simulink model "pi_IL_H2DF_2024a"  (R2024a)
settings: Solver=FixedStepAuto  StartTime=0.0  StopTime=inf  FixedStep=0.001  RelTol=1e-3  EnableMultiTasking=on
values from neighbouring files (symbols this model uses):
  IL = struct()    [init_simulink_IL_H2DF.m]
undefined symbols (not defined in the file or in its folder): C2C_NMPC
libraries: deeplib x1, raspberrypiNetworklib x1
(part 2 of 2)

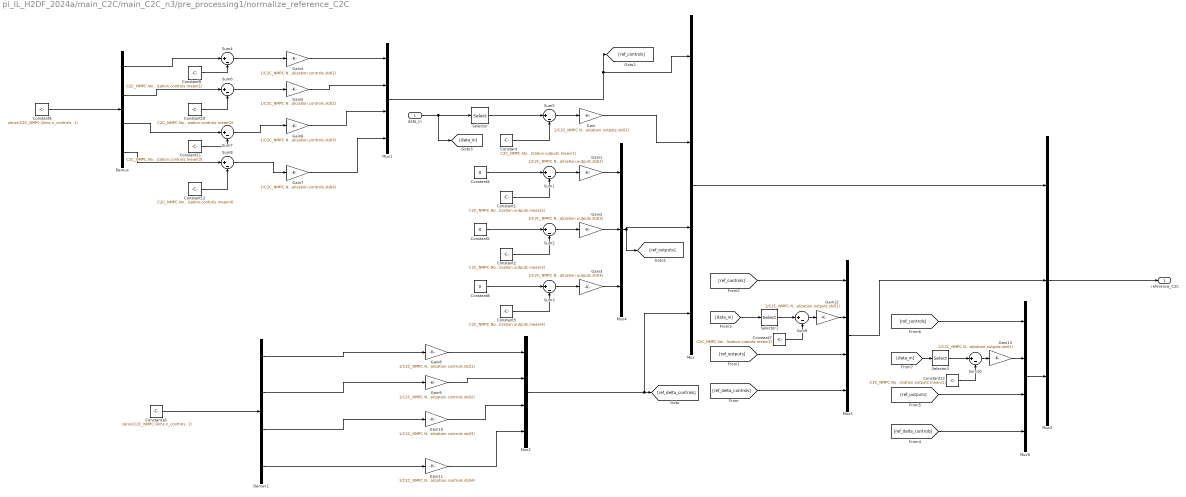
== system pi_IL_H2DF_2024a/main_C2C/main_C2C_n3/pre_processing1/normalize_reference_C2C ==
  data_in : Inport
  Constant : Constant  Value=C2C_NMPC.Normalization.outputs.mean(1)
  Constant1 : Constant  Value=C2C_NMPC.Normalization.outputs.mean(2)
  Constant10 : Constant  Value=C2C_NMPC.Normalization.controls.mean(2)
  Constant11 : Constant  Value=C2C_NMPC.Normalization.controls.mean(3)
  Constant12 : Constant  Value=C2C_NMPC.Normalization.controls.mean(4)
  Constant13 : Constant  Value=C2C_NMPC.Normalization.outputs.mean(1)
  Constant16 : Constant  Value=zeros(C2C_NMPC.Dims.n_controls, 1)
  Constant2 : Constant  Value=C2C_NMPC.Normalization.outputs.mean(3)
  Constant3 : Constant  Value=C2C_NMPC.Normalization.outputs.mean(4)
  Constant4 : Constant  Value=0
  Constant5 : Constant  Value=0
  Constant6 : Constant  Value=zeros(C2C_NMPC.Dims.n_controls, 1)
  Constant7 : Constant  Value=C2C_NMPC.Normalization.outputs.mean(1)
  Constant8 : Constant  Value=0
  Constant9 : Constant  Value=C2C_NMPC.Normalization.controls.mean(1)
  Demux : Demux
  Demux1 : Demux
  Gain : Gain  Gain=1/C2C_NMPC.Normalization.outputs.std(1)
  Gain1 : Gain  Gain=1/C2C_NMPC.Normalization.outputs.std(2)
  Gain10 : Gain  Gain=1/C2C_NMPC.Normalization.controls.std(3)
  Gain11 : Gain  Gain=1/C2C_NMPC.Normalization.controls.std(4)
  Gain12 : Gain  Gain=1/C2C_NMPC.Normalization.outputs.std(1)
  Gain13 : Gain  Gain=1/C2C_NMPC.Normalization.outputs.std(1)
  Gain2 : Gain  Gain=1/C2C_NMPC.Normalization.outputs.std(3)
  Gain3 : Gain  Gain=1/C2C_NMPC.Normalization.outputs.std(4)
  Gain4 : Gain  Gain=1/C2C_NMPC.Normalization.controls.std(1)
  Gain5 : Gain  Gain=1/C2C_NMPC.Normalization.controls.std(2)
  Gain6 : Gain  Gain=1/C2C_NMPC.Normalization.controls.std(3)
  Gain7 : Gain  Gain=1/C2C_NMPC.Normalization.controls.std(4)
  Gain8 : Gain  Gain=1/C2C_NMPC.Normalization.controls.std(1)
  Gain9 : Gain  Gain=1/C2C_NMPC.Normalization.controls.std(2)
  Mux{,1..2,5..6} (5 alike) : Mux
  Mux3 : Mux  Inputs=3
  Mux4 : Mux  Inputs=3
  Selector : Selector  IndexOptions=Index vector (dialog)  Indices=[5]  OutputSizes=1
  Selector1 : Selector  IndexOptions=Index vector (dialog)  Indices=7  OutputSizes=1
  Selector2 : Selector  IndexOptions=Index vector (dialog)  Indices=8  OutputSizes=1
  Sum{1..10} (10 alike) : Sum  Inputs=|+-
  reference_C2C : Outport  VectorParamsAs1DForOutWhenUnconnected=off
  wires:
  Constant/1 -> Sum5/2
  data_in/1 -> [data_in], Selector/1
  Sum5/1 -> Gain/1
  Selector/1 -> Sum5/1
  Constant4/1 -> Sum1/1
  Sum1/1 -> Gain1/1
  Constant1/1 -> Sum1/2
  Constant5/1 -> Sum2/1
  Sum2/1 -> Gain2/1
  Constant2/1 -> Sum2/2
  Constant8/1 -> Sum3/1
  Sum3/1 -> Gain3/1
  Constant3/1 -> Sum3/2
  Demux/1 -> Sum4/1
  Sum4/1 -> Gain4/1
  Constant9/1 -> Sum4/2
  Constant6/1 -> Demux/1
  Demux/2 -> Sum6/1
  Constant10/1 -> Sum6/2
  Sum6/1 -> Gain5/1
  Gain5/1 -> Mux1/2
  Gain4/1 -> Mux1/1
  Sum7/1 -> Gain6/1
  Constant11/1 -> Sum7/2
  Demux/3 -> Sum7/1
  Constant12/1 -> Sum8/2
  Sum8/1 -> Gain7/1
  Demux/4 -> Sum8/1
  Gain7/1 -> Mux1/4
  Gain6/1 -> Mux1/3
  Gain9/1 -> Mux2/2
  Gain11/1 -> Mux2/4
  Constant16/1 -> Demux1/1
  Gain8/1 -> Mux2/1
  Gain10/1 -> Mux2/3
  Demux1/4 -> Gain11/1
  Demux1/3 -> Gain10/1
  Demux1/2 -> Gain9/1
  Demux1/1 -> Gain8/1
  Mux2/1 -> [ref_delta_controls], Mux/4
  Mux3/1 -> reference_C2C/1
  Mux/1 -> Mux3/1
  Gain1/1 -> Mux4/1
  Gain2/1 -> Mux4/2
  Gain3/1 -> Mux4/3
  Gain/1 -> Mux/2
  Mux4/1 -> Mux/3, [ref_outputs]
  [ref_delta_controls] -> Mux5/4
  [ref_outputs] -> Mux5/3
  Mux1/1 -> [ref_controls], Mux/1
  [ref_controls] -> Mux5/1
  [data_in] -> Selector1/1
  Mux5/1 -> Mux3/2
  [data_in] -> Selector2/1
  [ref_controls] -> Mux6/1
  [ref_outputs] -> Mux6/3
  [ref_delta_controls] -> Mux6/4
  Mux6/1 -> Mux3/3
  Selector1/1 -> Sum9/1
  Sum9/1 -> Gain12/1
  Constant7/1 -> Sum9/2
  Gain12/1 -> Mux5/2
  Constant13/1 -> Sum10/2
  Sum10/1 -> Gain13/1
  Selector2/1 -> Sum10/1
  Gain13/1 -> Mux6/2

== system pi_IL_H2DF_2024a/main_C2C/main_C2C_n3/IL_Controller/IL_Controller_fb_FF_1/Denorm_NN_Controls ==
  controls_nn : Inport
  Constant4 : Constant  Value=IL.Normalization.outputs.mean(1)
  Constant5 : Constant  Value=IL.Normalization.outputs.mean(2)
  Constant6 : Constant  Value=IL.Normalization.outputs.mean(3)
  Constant7 : Constant  Value=IL.Normalization.outputs.mean(4)
  Demux : Demux
  Gain4 : Gain  Gain=IL.Normalization.outputs.std(1)
  Gain5 : Gain  Gain=IL.Normalization.outputs.std(2)
  Gain6 : Gain  Gain=IL.Normalization.outputs.std(3)
  Gain7 : Gain  Gain=IL.Normalization.outputs.std(4)
  Mux : Mux
  Sum{4,6..8} (4 alike) : Sum  Inputs=|++
  denorm_nn_u : Outport
  wires:
  Sum4/1 -> Mux/2
  Sum6/1 -> Mux/3
  controls_nn/1 -> Demux/1
  Demux/2 -> Gain5/1  "P2M"
  Demux/3 -> Gain6/1  "SOI_main"
  Demux/4 -> Gain7/1  "DOI_H2"
  Demux/1 -> Gain4/1  "DOI_main"
  Mux/1 -> denorm_nn_u/1
  Gain7/1 -> Sum7/1
  Gain6/1 -> Sum6/1
  Constant7/1 -> Sum7/2
  Constant5/1 -> Sum4/2
  Gain4/1 -> Sum8/1
  Gain5/1 -> Sum4/1
  Constant6/1 -> Sum6/2
  Constant4/1 -> Sum8/2
  Sum8/1 -> Mux/1
  Sum7/1 -> Mux/4

== system pi_IL_H2DF_2024a/main_C2C/main_C2C_n3/IL_Controller/IL_Controller_fb_FF_1/Norm_NN_IMEP_ref ==
  In : Inport
  Constant9 : Constant  Value=IL.Normalization.inputs.mean(1)
  Gain4 : Gain  Gain=1/IL.Normalization.inputs.std(1)
  Sum4 : Sum  Inputs=|+-
  Out : Outport
  wires:
  In/1 -> Sum4/1  "IMEP"
  Constant9/1 -> Sum4/2
  Sum4/1 -> Gain4/1
  Gain4/1 -> Out/1

== system pi_IL_H2DF_2024a/main_C2C/main_C2C_n3/IL_Controller/IL_Controller_fb_FF_1/Norm_NN_IMEP_ref1 ==
  In : Inport
  Constant9 : Constant  Value=IL.Normalization.inputs.mean(1)
  Gain4 : Gain  Gain=1/IL.Normalization.inputs.std(1)
  Sum4 : Sum  Inputs=|+-
  Out : Outport
  wires:
  Gain4/1 -> Out/1
  Sum4/1 -> Gain4/1
  Constant9/1 -> Sum4/2
  In/1 -> Sum4/1  "IMEP"

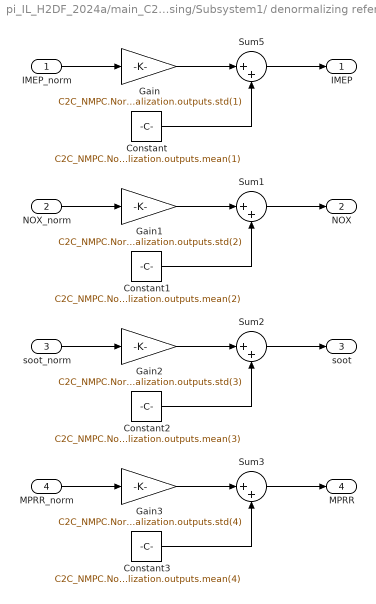
== system pi_IL_H2DF_2024a/main_C2C/main_C2C_n3/post_processing/Subsystem1/ denormalizing reference ==
  IMEP_norm : Inport
  NOX_norm : Inport  Port=2
  soot_norm : Inport  Port=3
  MPRR_norm : Inport  Port=4
  Constant : Constant  Value=C2C_NMPC.Normalization.outputs.mean(1)
  Constant1 : Constant  Value=C2C_NMPC.Normalization.outputs.mean(2)
  Constant2 : Constant  Value=C2C_NMPC.Normalization.outputs.mean(3)
  Constant3 : Constant  Value=C2C_NMPC.Normalization.outputs.mean(4)
  Gain : Gain  Gain=C2C_NMPC.Normalization.outputs.std(1)
  Gain1 : Gain  Gain=C2C_NMPC.Normalization.outputs.std(2)
  Gain2 : Gain  Gain=C2C_NMPC.Normalization.outputs.std(3)
  Gain3 : Gain  Gain=C2C_NMPC.Normalization.outputs.std(4)
  Sum{1..3,5} (4 alike) : Sum  Inputs=|++
  IMEP : Outport
  NOX : Outport  Port=2
  soot : Outport  Port=3
  MPRR : Outport  Port=4
  wires:
  Gain/1 -> Sum5/1
  IMEP_norm/1 -> Gain/1
  Constant/1 -> Sum5/2
  Sum5/1 -> IMEP/1
  Gain1/1 -> Sum1/1
  Constant1/1 -> Sum1/2
  NOX_norm/1 -> Gain1/1
  Sum1/1 -> NOX/1
  Gain2/1 -> Sum2/1
  Constant2/1 -> Sum2/2
  soot_norm/1 -> Gain2/1
  Sum2/1 -> soot/1
  Gain3/1 -> Sum3/1
  Constant3/1 -> Sum3/2
  MPRR_norm/1 -> Gain3/1
  Sum3/1 -> MPRR/1

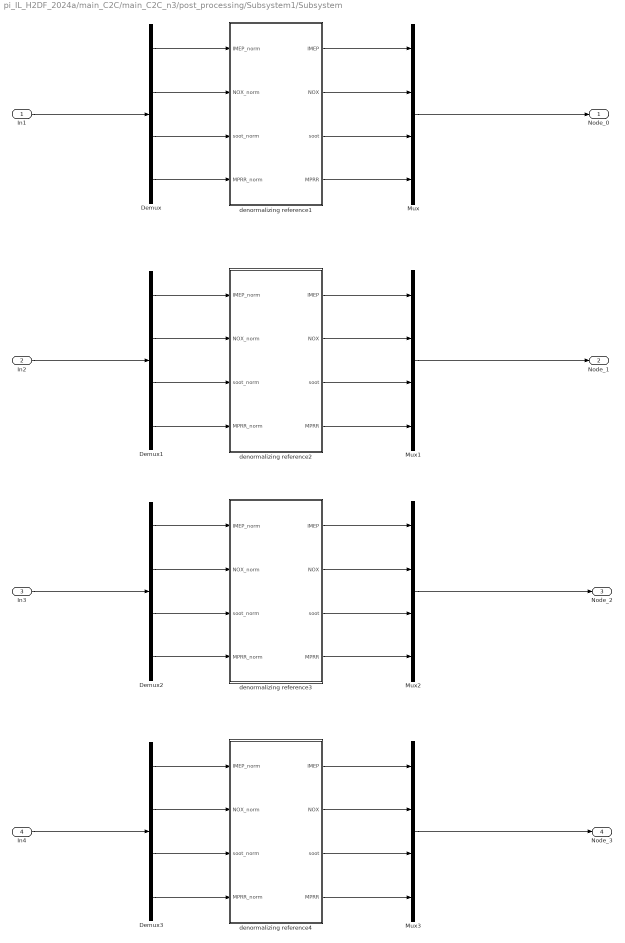
== system pi_IL_H2DF_2024a/main_C2C/main_C2C_n3/post_processing/Subsystem1/Subsystem ==
  In1 : Inport
  In2 : Inport  Port=2
  In3 : Inport  Port=3
  In4 : Inport  Port=4
  " denormalizing reference1" : Subsystem
  " denormalizing reference2" : Subsystem
  " denormalizing reference3" : Subsystem
  " denormalizing reference4" : Subsystem
  Demux{,1..3} (4 alike) : Demux
  Mux{,1..3} (4 alike) : Mux
  Node_0 : Outport
  Node_1 : Outport  Port=2
  Node_2 : Outport  Port=3
  Node_3 : Outport  Port=4
  wires:
  Demux/1 -> " denormalizing reference1"/1(IMEP_norm)
  Demux/2 -> " denormalizing reference1"/2(NOX_norm)
  Demux/3 -> " denormalizing reference1"/3(soot_norm)
  Demux/4 -> " denormalizing reference1"/4(MPRR_norm)
  In1/1 -> Demux/1
  " denormalizing reference1"/1(IMEP) -> Mux/1
  " denormalizing reference1"/2(NOX) -> Mux/2
  " denormalizing reference1"/3(soot) -> Mux/3
  " denormalizing reference1"/4(MPRR) -> Mux/4
  " denormalizing reference2"/3(soot) -> Mux1/3
  Demux1/3 -> " denormalizing reference2"/3(soot_norm)
  In2/1 -> Demux1/1
  " denormalizing reference2"/2(NOX) -> Mux1/2
  " denormalizing reference2"/1(IMEP) -> Mux1/1
  Demux1/1 -> " denormalizing reference2"/1(IMEP_norm)
  Demux1/4 -> " denormalizing reference2"/4(MPRR_norm)
  Demux1/2 -> " denormalizing reference2"/2(NOX_norm)
  " denormalizing reference2"/4(MPRR) -> Mux1/4
  " denormalizing reference3"/3(soot) -> Mux2/3
  Demux2/3 -> " denormalizing reference3"/3(soot_norm)
  In3/1 -> Demux2/1
  " denormalizing reference3"/2(NOX) -> Mux2/2
  " denormalizing reference3"/1(IMEP) -> Mux2/1
  Demux2/1 -> " denormalizing reference3"/1(IMEP_norm)
  Demux2/4 -> " denormalizing reference3"/4(MPRR_norm)
  Demux2/2 -> " denormalizing reference3"/2(NOX_norm)
  " denormalizing reference3"/4(MPRR) -> Mux2/4
  " denormalizing reference4"/3(soot) -> Mux3/3
  Demux3/3 -> " denormalizing reference4"/3(soot_norm)
  In4/1 -> Demux3/1
  " denormalizing reference4"/2(NOX) -> Mux3/2
  " denormalizing reference4"/1(IMEP) -> Mux3/1
  Demux3/1 -> " denormalizing reference4"/1(IMEP_norm)
  Demux3/4 -> " denormalizing reference4"/4(MPRR_norm)
  Demux3/2 -> " denormalizing reference4"/2(NOX_norm)
  " denormalizing reference4"/4(MPRR) -> Mux3/4
  Mux/1 -> Node_0/1
  Mux1/1 -> Node_1/1
  Mux2/1 -> Node_2/1
  Mux3/1 -> Node_3/1

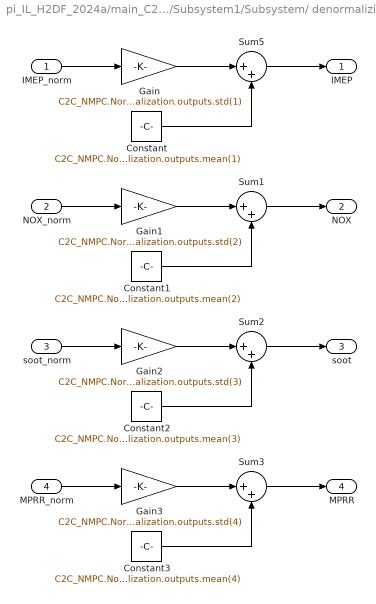
== system pi_IL_H2DF_2024a/main_C2C/main_C2C_n3/post_processing/Subsystem1/Subsystem/ denormalizing reference1 ==
  IMEP_norm : Inport
  NOX_norm : Inport  Port=2
  soot_norm : Inport  Port=3
  MPRR_norm : Inport  Port=4
  Constant : Constant  Value=C2C_NMPC.Normalization.outputs.mean(1)
  Constant1 : Constant  Value=C2C_NMPC.Normalization.outputs.mean(2)
  Constant2 : Constant  Value=C2C_NMPC.Normalization.outputs.mean(3)
  Constant3 : Constant  Value=C2C_NMPC.Normalization.outputs.mean(4)
  Gain : Gain  Gain=C2C_NMPC.Normalization.outputs.std(1)
  Gain1 : Gain  Gain=C2C_NMPC.Normalization.outputs.std(2)
  Gain2 : Gain  Gain=C2C_NMPC.Normalization.outputs.std(3)
  Gain3 : Gain  Gain=C2C_NMPC.Normalization.outputs.std(4)
  Sum{1..3,5} (4 alike) : Sum  Inputs=|++
  IMEP : Outport
  NOX : Outport  Port=2
  soot : Outport  Port=3
  MPRR : Outport  Port=4
  wires:
  Gain/1 -> Sum5/1
  IMEP_norm/1 -> Gain/1
  Constant/1 -> Sum5/2
  Sum5/1 -> IMEP/1
  Gain1/1 -> Sum1/1
  Constant1/1 -> Sum1/2
  NOX_norm/1 -> Gain1/1
  Sum1/1 -> NOX/1
  Gain2/1 -> Sum2/1
  Constant2/1 -> Sum2/2
  soot_norm/1 -> Gain2/1
  Sum2/1 -> soot/1
  Gain3/1 -> Sum3/1
  Constant3/1 -> Sum3/2
  MPRR_norm/1 -> Gain3/1
  Sum3/1 -> MPRR/1

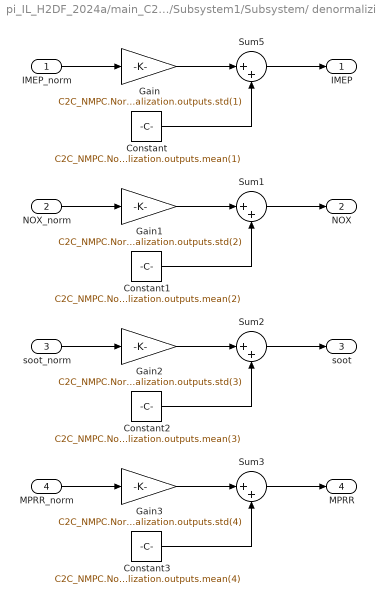
== system pi_IL_H2DF_2024a/main_C2C/main_C2C_n3/post_processing/Subsystem1/Subsystem/ denormalizing reference2 ==
  IMEP_norm : Inport
  NOX_norm : Inport  Port=2
  soot_norm : Inport  Port=3
  MPRR_norm : Inport  Port=4
  Constant : Constant  Value=C2C_NMPC.Normalization.outputs.mean(1)
  Constant1 : Constant  Value=C2C_NMPC.Normalization.outputs.mean(2)
  Constant2 : Constant  Value=C2C_NMPC.Normalization.outputs.mean(3)
  Constant3 : Constant  Value=C2C_NMPC.Normalization.outputs.mean(4)
  Gain : Gain  Gain=C2C_NMPC.Normalization.outputs.std(1)
  Gain1 : Gain  Gain=C2C_NMPC.Normalization.outputs.std(2)
  Gain2 : Gain  Gain=C2C_NMPC.Normalization.outputs.std(3)
  Gain3 : Gain  Gain=C2C_NMPC.Normalization.outputs.std(4)
  Sum{1..3,5} (4 alike) : Sum  Inputs=|++
  IMEP : Outport
  NOX : Outport  Port=2
  soot : Outport  Port=3
  MPRR : Outport  Port=4
  wires:
  Gain/1 -> Sum5/1
  IMEP_norm/1 -> Gain/1
  Constant/1 -> Sum5/2
  Sum5/1 -> IMEP/1
  Gain1/1 -> Sum1/1
  Constant1/1 -> Sum1/2
  NOX_norm/1 -> Gain1/1
  Sum1/1 -> NOX/1
  Gain2/1 -> Sum2/1
  Constant2/1 -> Sum2/2
  soot_norm/1 -> Gain2/1
  Sum2/1 -> soot/1
  Gain3/1 -> Sum3/1
  Constant3/1 -> Sum3/2
  MPRR_norm/1 -> Gain3/1
  Sum3/1 -> MPRR/1

== system pi_IL_H2DF_2024a/main_C2C/main_C2C_n3/post_processing/Subsystem1/Subsystem/ denormalizing reference3 ==
  IMEP_norm : Inport
  NOX_norm : Inport  Port=2
  soot_norm : Inport  Port=3
  MPRR_norm : Inport  Port=4
  Constant : Constant  Value=C2C_NMPC.Normalization.outputs.mean(1)
  Constant1 : Constant  Value=C2C_NMPC.Normalization.outputs.mean(2)
  Constant2 : Constant  Value=C2C_NMPC.Normalization.outputs.mean(3)
  Constant3 : Constant  Value=C2C_NMPC.Normalization.outputs.mean(4)
  Gain : Gain  Gain=C2C_NMPC.Normalization.outputs.std(1)
  Gain1 : Gain  Gain=C2C_NMPC.Normalization.outputs.std(2)
  Gain2 : Gain  Gain=C2C_NMPC.Normalization.outputs.std(3)
  Gain3 : Gain  Gain=C2C_NMPC.Normalization.outputs.std(4)
  Sum{1..3,5} (4 alike) : Sum  Inputs=|++
  IMEP : Outport
  NOX : Outport  Port=2
  soot : Outport  Port=3
  MPRR : Outport  Port=4
  wires:
  Gain/1 -> Sum5/1
  IMEP_norm/1 -> Gain/1
  Constant/1 -> Sum5/2
  Sum5/1 -> IMEP/1
  Gain1/1 -> Sum1/1
  Constant1/1 -> Sum1/2
  NOX_norm/1 -> Gain1/1
  Sum1/1 -> NOX/1
  Gain2/1 -> Sum2/1
  Constant2/1 -> Sum2/2
  soot_norm/1 -> Gain2/1
  Sum2/1 -> soot/1
  Gain3/1 -> Sum3/1
  Constant3/1 -> Sum3/2
  MPRR_norm/1 -> Gain3/1
  Sum3/1 -> MPRR/1

== system pi_IL_H2DF_2024a/main_C2C/main_C2C_n3/post_processing/Subsystem1/Subsystem/ denormalizing reference4 ==
  IMEP_norm : Inport
  NOX_norm : Inport  Port=2
  soot_norm : Inport  Port=3
  MPRR_norm : Inport  Port=4
  Constant : Constant  Value=C2C_NMPC.Normalization.outputs.mean(1)
  Constant1 : Constant  Value=C2C_NMPC.Normalization.outputs.mean(2)
  Constant2 : Constant  Value=C2C_NMPC.Normalization.outputs.mean(3)
  Constant3 : Constant  Value=C2C_NMPC.Normalization.outputs.mean(4)
  Gain : Gain  Gain=C2C_NMPC.Normalization.outputs.std(1)
  Gain1 : Gain  Gain=C2C_NMPC.Normalization.outputs.std(2)
  Gain2 : Gain  Gain=C2C_NMPC.Normalization.outputs.std(3)
  Gain3 : Gain  Gain=C2C_NMPC.Normalization.outputs.std(4)
  Sum{1..3,5} (4 alike) : Sum  Inputs=|++
  IMEP : Outport
  NOX : Outport  Port=2
  soot : Outport  Port=3
  MPRR : Outport  Port=4
  wires:
  Gain/1 -> Sum5/1
  IMEP_norm/1 -> Gain/1
  Constant/1 -> Sum5/2
  Sum5/1 -> IMEP/1
  Gain1/1 -> Sum1/1
  Constant1/1 -> Sum1/2
  NOX_norm/1 -> Gain1/1
  Sum1/1 -> NOX/1
  Gain2/1 -> Sum2/1
  Constant2/1 -> Sum2/2
  soot_norm/1 -> Gain2/1
  Sum2/1 -> soot/1
  Gain3/1 -> Sum3/1
  Constant3/1 -> Sum3/2
  MPRR_norm/1 -> Gain3/1
  Sum3/1 -> MPRR/1

== stateflow chart pi_IL_H2DF_2024a/Chart1 ==
  state wait
  (default) -> wait
  wait -> (junction 9) : [size>0]{call_main_C2C; call_tx_C2C}
  (junction 10) -> wait
  (junction 9) -> (junction 10)
  data: size input
  events: call_tx_C2C output FUNCTION_CALL_EVENT; call_main_C2C output FUNCTION_CALL_EVENT
